simulink model "MBD_Week3_Prob1"  (R2020a)
settings: Solver=VariableStepAuto  StartTime=0.0  StopTime=inf  RelTol=1e-3
settings Model: EnablePacing=on  PacingRate=0.089000  Creator=Noel Varghese  LastModifiedBy=Noel Varghese

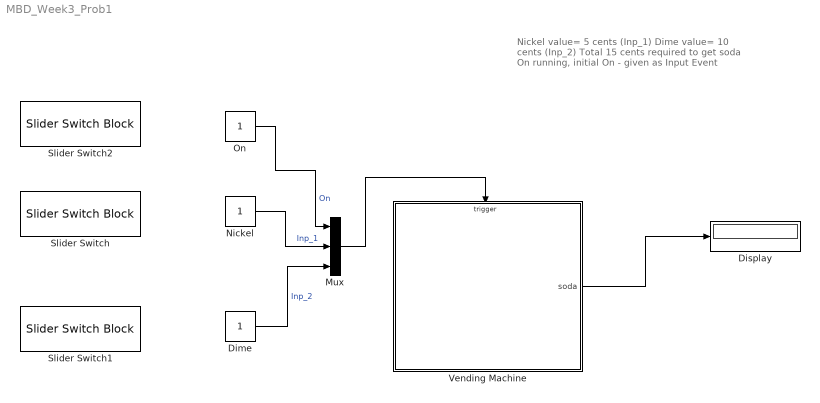
== system MBD_Week3_Prob1 ==
  note: Nickel value= 5 cents (Inp_1)
      | Dime value= 10 cents (Inp_2)
      | Total 15 cents required to get soda
      | On running, initial On - given as Input Event
  Dime : Constant
  Display : Display
  Mux : Mux  Inputs=3
  Nickel : Constant
  On : Constant
  Slider Switch : SliderSwitchBlock
      settings: Values={{'Off', 'On'}, [0 1]}
  Slider Switch1 : SliderSwitchBlock
      settings: Values={{'Off', 'On'}, [0 1]}
  Slider Switch2 : SliderSwitchBlock
      settings: Values={{'Off', 'On'}, [0 1]}
  Vending Machine : Stateflow chart  TreatAsAtomicUnit=on
  wires:
  Vending Machine/1(soda) -> Display/1
  Mux/1 -> Vending Machine/Trigger
  Nickel/1 -> Mux/2  "Inp_1"
  Dime/1 -> Mux/3  "Inp_2"
  On/1 -> Mux/1  "On"

== stateflow chart MBD_Week3_Prob1/Vending Machine ==
  note: Nickel value= 5 cents (Inp_1)
      | Dime value= 10 cents (Inp_2)
      | Total 15 cents required to get soda
  state coin_zero
  state coin_dime
  state coin_nickel
  (default) -> coin_zero
  coin_nickel -> coin_zero [order 2] : Inp_2{soda=1}
  coin_zero -> coin_dime [order 2] : Inp_2{soda=0}
  coin_dime -> coin_zero [order 1] : Inp_1{soda=1}
  coin_zero -> coin_nickel [order 1] : Inp_1{soda=0}
  coin_dime -> coin_nickel [order 2] : Inp_2{soda=1}
  coin_nickel -> coin_dime [order 1] : Inp_1{soda=0}
  data: soda output
  events: Input_Event input EITHER_EDGE_EVENT; Inp_1 input EITHER_EDGE_EVENT; Inp_2 input EITHER_EDGE_EVENT
